simulink model "airspeed_controller16b"  (R2016b)
settings: Solver=FixedStepAuto  StartTime=0.0  StopTime=1000  FixedStep=0.001  RelTol=1e-3
model workspace (MAT data in the model file):
  Cd = 0.18
  SBE_rate_pitch = 0
  climb_max = 5
  g_common = 9.81
  mass_plane = 1.5
  nomThr = 0
  pitch_damping_gain = 0
  pitch_integ_gain = 0.1
  pitch_time_constant = 5
  rou = 1.225
  sink_max = 1
  timeConstThrot = 8
libraries: simulink x2
settings Model: Creator=lee  LastModifiedBy=ls
settings SFSimCC: SimUseLocalCustomCode=on
settings RTWCC: RTWUseLocalCustomCode=on

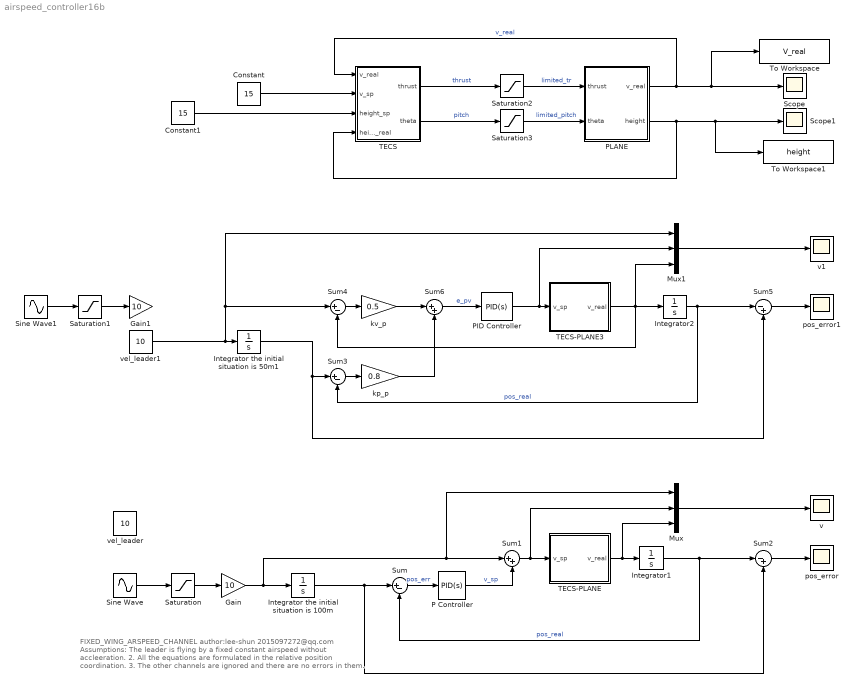
== system airspeed_controller16b ==
  note: FIXED_WING_ARSPEED_CHANNEL
      |
      | author:lee-shun 2015097272@qq.com
      |
      | Assumptions:
      |
      | The leader is flying by a fixed constant airspeed without accleeration.
      | 2. All the equations are formulated in the relative position coordination.
      | 3. The other channels are ignored and there are no errors in them.
  Constant : Constant  Value=15
  Constant1 : Constant  Value=15
  Gain : Gain  Gain=10
  Gain1 : Gain  Gain=10
  Integrator the initial situation is 100m : Integrator  InitialCondition=50  IgnoreLimit=on
  Integrator the initial situation is 50m1 : Integrator  InitialCondition=50  IgnoreLimit=on
  Integrator1 : Integrator
  Integrator2 : Integrator
  Mux : Mux  Inputs=3
  Mux1 : Mux  Inputs=3
  P Controller : simulink/Continuous/PID Controller  Controller=PID  Form=Parallel  TimeDomain=Continuous-time  SampleTime=-1  IntegratorMethod=Forward Euler  FilterMethod=Forward Euler  ControllerParametersSource=internal  P=0.02  I=0  D=0.0  UseFilter=on  N=100  InitialConditionSource=internal  InitialConditionForIntegrator=0  InitialConditionForFilter=0  DifferentiatorICPrevScaledInput=0  ExternalReset=none  TrackingMode=off  Kt=1  LimitOutput=off  UpperSaturationLimit=inf  LowerSaturationLimit=-inf  LinearizeAsGain=on  AntiWindupMode=none  Kb=1  POutMin=[]  POutMax=[]  IOutMin=[]  IOutMax=[]  DOutMin=[]  DOutMax=[]  NOutMin=[]  NOutMax=[]  SumOutMin=[]  SumOutMax=[]  SaturationOutMin=[]  SaturationOutMax=[]  PParamMin=[]  PParamMax=[]  IParamMin=[]  IParamMax=[]  DParamMin=[]  DParamMax=[]  NParamMin=[]  NParamMax=[]  KbParamMin=[]  KbParamMax=[]  KtParamMin=[]  KtParamMax=[]  KbOutMin=[]  KbOutMax=[]  KtOutMin=[]  KtOutMax=[]  IntegratorOutMin=[]  IntegratorOutMax=[]  FilterOutMin=[]  FilterOutMax=[]  SumI1OutMin=[]  SumI1OutMax=[]  SumI2OutMin=[]  SumI2OutMax=[]  SumI3OutMin=[]  SumI3OutMax=[]  SumDOutMin=[]  SumDOutMax=[]  DifferentiatorOutMin=[]  DifferentiatorOutMax=[]  IntegratorContinuousStateAttributes=''  IntegratorStateMustResolveToSignalObject=off  IntegratorRTWStateStorageClass=Auto  FilterContinuousStateAttributes=''  FilterStateMustResolveToSignalObject=off  FilterRTWStateStorageClass=Auto
  PID Controller : simulink/Continuous/PID Controller  Controller=PID  Form=Parallel  TimeDomain=Continuous-time  SampleTime=-1  IntegratorMethod=Forward Euler  FilterMethod=Forward Euler  ControllerParametersSource=internal  P=0.3  I=0.01  D=0  UseFilter=on  N=100  InitialConditionSource=internal  InitialConditionForIntegrator=0  InitialConditionForFilter=0  DifferentiatorICPrevScaledInput=0  ExternalReset=none  TrackingMode=off  Kt=1  LimitOutput=off  UpperSaturationLimit=inf  LowerSaturationLimit=-inf  LinearizeAsGain=on  AntiWindupMode=none  Kb=1  POutMin=[]  POutMax=[]  IOutMin=[]  IOutMax=[]  DOutMin=[]  DOutMax=[]  NOutMin=[]  NOutMax=[]  SumOutMin=[]  SumOutMax=[]  SaturationOutMin=[]  SaturationOutMax=[]  PParamMin=[]  PParamMax=[]  IParamMin=[]  IParamMax=[]  DParamMin=[]  DParamMax=[]  NParamMin=[]  NParamMax=[]  KbParamMin=[]  KbParamMax=[]  KtParamMin=[]  KtParamMax=[]  KbOutMin=[]  KbOutMax=[]  KtOutMin=[]  KtOutMax=[]  IntegratorOutMin=[]  IntegratorOutMax=[]  FilterOutMin=[]  FilterOutMax=[]  SumI1OutMin=[]  SumI1OutMax=[]  SumI2OutMin=[]  SumI2OutMax=[]  SumI3OutMin=[]  SumI3OutMax=[]  SumDOutMin=[]  SumDOutMax=[]  DifferentiatorOutMin=[]  DifferentiatorOutMax=[]  IntegratorContinuousStateAttributes=''  IntegratorStateMustResolveToSignalObject=off  IntegratorRTWStateStorageClass=Auto  FilterContinuousStateAttributes=''  FilterStateMustResolveToSignalObject=off  FilterRTWStateStorageClass=Auto
  PLANE : Subsystem
  Saturation : Saturate  UpperLimit=1  LowerLimit=0.2
  Saturation1 : Saturate  UpperLimit=1  LowerLimit=0.2
  Saturation2 : Saturate  UpperLimit=1  LowerLimit=0  ZeroCross=off
  Saturation3 : Saturate  UpperLimit=pi/4  LowerLimit=-pi/6  ZeroCross=off
  Scope : Scope
  Scope1 : Scope
  Sine Wave : Sin  Frequency=0.1  SampleTime=0
  Sine Wave1 : Sin  Frequency=0.1  SampleTime=0
  Sum : Sum  Inputs=|+-
  Sum1 : Sum  Inputs=|++
  Sum2 : Sum  Inputs=|-+
  Sum3 : Sum  Inputs=|+-
  Sum4 : Sum  Inputs=|+-
  Sum5 : Sum  Inputs=|-+
  Sum6 : Sum  Inputs=|++
  "TECS " : Subsystem
  TECS-PLANE : Subsystem
  TECS-PLANE3 : Subsystem
  To Workspace : ToWorkspace  VariableName=V_real  SaveFormat=Timeseries  SampleTime=-1
  To Workspace1 : ToWorkspace  VariableName=height  SaveFormat=Timeseries  SampleTime=-1
  kp_p : Gain  Gain=0.8
  kv_p : Gain  Gain=0.5
  pos_error : Scope
  pos_error1 : Scope
  v : Scope
  v1 : Scope
  vel_leader : Constant  Value=10
  vel_leader1 : Constant  Value=10
  wires:
  Sum/1 -> P Controller/1  "pos_err"
  Integrator1/1 -> Sum/2, Sum2/1  "pos_real"
  Integrator the initial situation is 100m/1 -> Sum/1, Sum2/2
  TECS-PLANE/1(v_real) -> Mux/3, Integrator1/1
  P Controller/1 -> Sum1/2  "v_sp"
  Sum1/1 -> Mux/2, TECS-PLANE/1(v_sp)
  Sum2/1 -> pos_error/1
  Sine Wave/1 -> Saturation/1
  Saturation/1 -> Gain/1
  Gain/1 -> Mux/1, Sum1/1, Integrator the initial situation is 100m/1
  Mux/1 -> v/1
  Sum5/1 -> pos_error1/1
  Saturation1/1 -> Gain1/1
  Sine Wave1/1 -> Saturation1/1
  TECS-PLANE3/1(v_real) -> Integrator2/1, Mux1/3, Sum4/2
  Integrator2/1 -> Sum5/1, Sum3/2  "pos_real"
  Mux1/1 -> v1/1
  Integrator the initial situation is 50m1/1 -> Sum3/1, Sum5/2
  kv_p/1 -> Sum6/1
  Sum4/1 -> kv_p/1
  Sum3/1 -> kp_p/1
  kp_p/1 -> Sum6/2
  Sum6/1 -> PID Controller/1  "e_pv"
  PID Controller/1 -> TECS-PLANE3/1(v_sp), Mux1/2
  vel_leader1/1 -> Sum4/1, Mux1/1, Integrator the initial situation is 50m1/1
  "TECS "/2("theta ") -> Saturation3/1  "pitch"
  PLANE/1(v_real) -> To Workspace/1, Scope/1, "TECS "/1(v_real)  "v_real"
  PLANE/2(height) -> To Workspace1/1, Scope1/1, "TECS "/4(height_real)
  Saturation3/1 -> PLANE/2(theta)  "limited_pitch"
  Constant/1 -> "TECS "/2(v_sp)
  "TECS "/1(thrust) -> Saturation2/1  "thrust"
  Saturation2/1 -> PLANE/1(thrust)  "limited_tr"
  Constant1/1 -> "TECS "/3(height_sp)

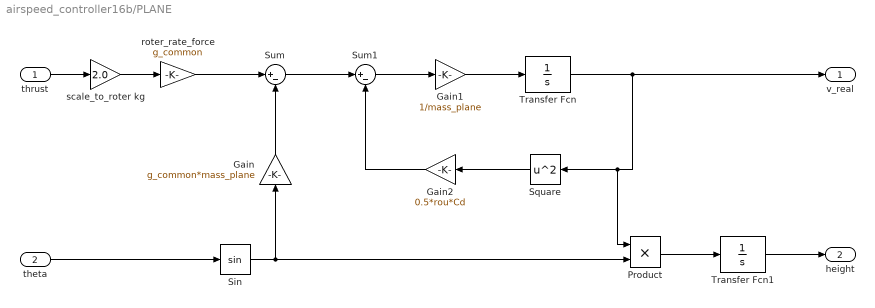
== system airspeed_controller16b/PLANE ==
  thrust : Inport
  theta : Inport  Port=2
  Gain : Gain  Gain=g_common*mass_plane
  Gain1 : Gain  Gain=1/mass_plane
  Gain2 : Gain  Gain=0.5*rou*Cd
  Product : Product
  Sin : Trigonometry
  Square : Math  Operator=square  SaturateOnIntegerOverflow=on
  Sum : Sum  Inputs=|+-
  Sum1 : Sum  Inputs=|+-
  Transfer Fcn : TransferFcn  Denominator=[1 0]
  Transfer Fcn1 : TransferFcn  Denominator=[1 0]
  roter_rate_force : Gain  Gain=g_common
  scale_to_roter kg : Gain  Gain=2.0
  v_real : Outport
  height : Outport  Port=2
  wires:
  thrust/1 -> scale_to_roter kg/1
  scale_to_roter kg/1 -> roter_rate_force/1
  roter_rate_force/1 -> Sum/1
  Gain/1 -> Sum/2
  theta/1 -> Sin/1
  Sin/1 -> Product/2, Gain/1
  Sum/1 -> Sum1/1
  Sum1/1 -> Gain1/1
  Gain1/1 -> Transfer Fcn/1
  Transfer Fcn/1 -> Product/1, Square/1, v_real/1
  Square/1 -> Gain2/1
  Gain2/1 -> Sum1/2
  Product/1 -> Transfer Fcn1/1
  Transfer Fcn1/1 -> height/1

== system airspeed_controller16b/TECS  ==
  v_real : Inport
  v_sp : Inport  Port=2
  height_sp : Inport  Port=3
  height_real : Inport  Port=4
  SBE : Subsystem
  STE : Subsystem
  Subsystem : Subsystem
  Subsystem1 : Subsystem
  Subsystem2 : Subsystem
  thrust : Outport
  "theta " : Outport  Port=2
  wires:
  v_sp/1 -> Subsystem/2(v_sp)
  v_real/1 -> Subsystem2/5(vel_real), Subsystem/1(v_real)
  height_sp/1 -> Subsystem/3(height_sp)
  height_real/1 -> Subsystem/4(height_real)
  Subsystem/1(SPE_sp) -> SBE/1(SPE_sp), STE/1(SPE_sp)
  Subsystem/2(SKE_sp) -> SBE/2(SKE_sp), STE/2(SKE_sp)
  Subsystem/3(SPE_rate_sp) -> SBE/3(SPE_rate_sp), STE/3(SPE_rate_sp)
  Subsystem/4(SKE_rate_sp) -> SBE/4(SKE_rate_sp), STE/4(SKE_rate_sp)
  Subsystem/6(SPE_real) -> SBE/6(SPE_real), STE/6(SPE_real)
  Subsystem/5(SKE_real) -> SBE/5(SKE_real), STE/5(SKE_real)
  Subsystem/7(SKE_rate_real) -> SBE/7(SKE_rate_real), STE/7(SKE_rate_real)
  Subsystem/8(SPE_rate_real) -> SBE/8(SPE_rate_real), STE/8(SPE_rate_real)
  STE/1(STE_real) -> Subsystem1/1(In1)
  STE/2(STE_sp) -> Subsystem1/2(In2)
  STE/3(STE_rate_real) -> Subsystem1/3(In3)
  STE/4(STE_rate_sp) -> Subsystem1/4(In4)
  Subsystem1/1(Out1) -> thrust/1
  SBE/1(SBE_real) -> Subsystem2/1(SBE_real)
  SBE/2(SBE_sp) -> Subsystem2/2(SBE_sp)
  SBE/3(SBE_rate_real) -> Subsystem2/3(SEB_rate_real)
  SBE/4(SBE_rate_sp) -> Subsystem2/4(SEB_rate_sp)
  Subsystem2/1(theta) -> "theta "/1

== system airspeed_controller16b/TECS-PLANE ==
  v_sp : Inport
  PLANE : Subsystem
  Saturation : Saturate  UpperLimit=1  LowerLimit=0  ZeroCross=off
  Scope : Scope
  "TECS " : Subsystem
  v_real : Outport
  wires:
  PLANE/1(v_real) -> v_real/1, "TECS "/2(v_real)  "v_real"
  Saturation/1 -> Scope/1, PLANE/1(thrust)  "limited_tr"
  "TECS "/1(thrust) -> Saturation/1  "thrust"
  v_sp/1 -> "TECS "/1(v_sp)

== system airspeed_controller16b/TECS-PLANE3 ==
  v_sp : Inport
  PLANE : Subsystem
  Saturation : Saturate  UpperLimit=1  LowerLimit=0  ZeroCross=off
  Scope : Scope
  "TECS " : Subsystem
  Zero-Order Hold : ZeroOrderHold  SampleTime=-1
  v_real : Outport
  wires:
  PLANE/1(v_real) -> v_real/1, "TECS "/2(v_real)  "v_real"
  Saturation/1 -> Scope/1, PLANE/1(thrust)  "limited_tr"
  "TECS "/1(thrust) -> Zero-Order Hold/1  "thrust"
  v_sp/1 -> "TECS "/1(v_sp)
  Zero-Order Hold/1 -> Saturation/1

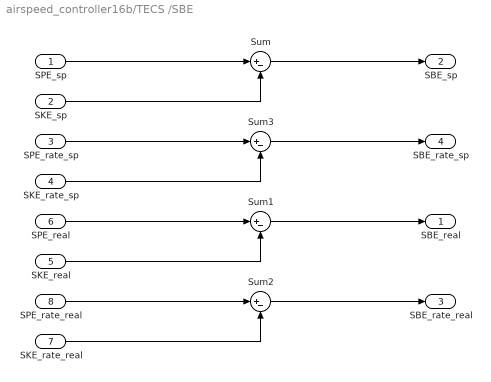
== system airspeed_controller16b/TECS /SBE ==
  SPE_sp : Inport
  SKE_sp : Inport  Port=2
  SPE_rate_sp : Inport  Port=3
  SKE_rate_sp : Inport  Port=4
  SKE_real : Inport  Port=5
  SPE_real : Inport  Port=6
  SKE_rate_real : Inport  Port=7
  SPE_rate_real : Inport  Port=8
  Sum{,1..3} (4 alike) : Sum  Inputs=|+-
  SBE_real : Outport
  SBE_sp : Outport  Port=2
  SBE_rate_real : Outport  Port=3
  SBE_rate_sp : Outport  Port=4
  wires:
  SKE_rate_sp/1 -> Sum3/2
  SKE_sp/1 -> Sum/2
  SPE_rate_sp/1 -> Sum3/1
  SPE_sp/1 -> Sum/1
  Sum/1 -> SBE_sp/1
  SPE_real/1 -> Sum1/1
  SKE_real/1 -> Sum1/2
  Sum1/1 -> SBE_real/1
  Sum3/1 -> SBE_rate_sp/1
  Sum2/1 -> SBE_rate_real/1
  SPE_rate_real/1 -> Sum2/1
  SKE_rate_real/1 -> Sum2/2

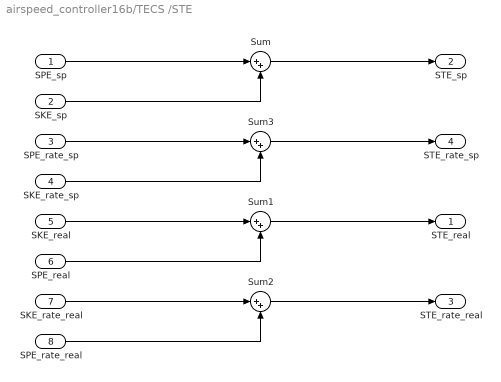
== system airspeed_controller16b/TECS /STE ==
  SPE_sp : Inport
  SKE_sp : Inport  Port=2
  SPE_rate_sp : Inport  Port=3
  SKE_rate_sp : Inport  Port=4
  SKE_real : Inport  Port=5
  SPE_real : Inport  Port=6
  SKE_rate_real : Inport  Port=7
  SPE_rate_real : Inport  Port=8
  Sum{,1..3} (4 alike) : Sum  Inputs=|++
  STE_real : Outport
  STE_sp : Outport  Port=2
  STE_rate_real : Outport  Port=3
  STE_rate_sp : Outport  Port=4
  wires:
  SPE_sp/1 -> Sum/1
  SKE_sp/1 -> Sum/2
  Sum/1 -> STE_sp/1
  SKE_real/1 -> Sum1/1
  Sum1/1 -> STE_real/1
  SPE_real/1 -> Sum1/2
  SKE_rate_real/1 -> Sum2/1
  Sum2/1 -> STE_rate_real/1
  SPE_rate_real/1 -> Sum2/2
  SPE_rate_sp/1 -> Sum3/1
  Sum3/1 -> STE_rate_sp/1
  SKE_rate_sp/1 -> Sum3/2

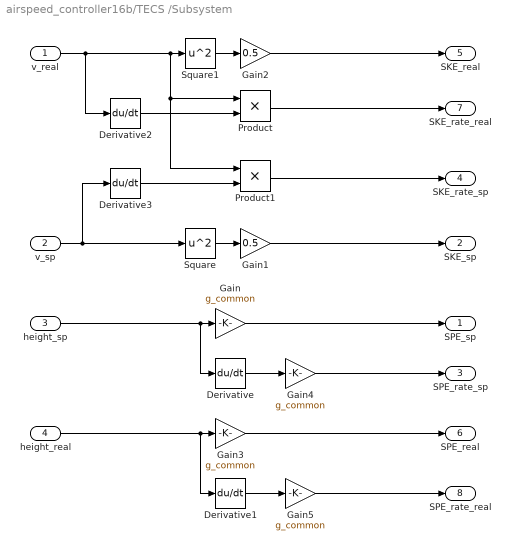
== system airspeed_controller16b/TECS /Subsystem ==
  v_real : Inport
  v_sp : Inport  Port=2
  height_sp : Inport  Port=3
  height_real : Inport  Port=4
  Derivative{,1..3} (4 alike) : Derivative
  Gain{,3..5} (4 alike) : Gain  Gain=g_common
  Gain1 : Gain  Gain=0.5
  Gain2 : Gain  Gain=0.5
  Product : Product
  Product1 : Product
  Square : Math  Operator=square  SaturateOnIntegerOverflow=on
  Square1 : Math  Operator=square  SaturateOnIntegerOverflow=on
  SPE_sp : Outport
  SKE_sp : Outport  Port=2
  SPE_rate_sp : Outport  Port=3
  SKE_rate_sp : Outport  Port=4
  SKE_real : Outport  Port=5
  SPE_real : Outport  Port=6
  SKE_rate_real : Outport  Port=7
  SPE_rate_real : Outport  Port=8
  wires:
  Gain/1 -> SPE_sp/1
  height_sp/1 -> Derivative/1, Gain/1
  Gain1/1 -> SKE_sp/1
  v_sp/1 -> Square/1, Derivative3/1
  Square/1 -> Gain1/1
  Square1/1 -> Gain2/1
  v_real/1 -> Product1/1, Product/1, Square1/1, Derivative2/1
  Gain2/1 -> SKE_real/1
  height_real/1 -> Derivative1/1, Gain3/1
  Gain3/1 -> SPE_real/1
  Gain4/1 -> SPE_rate_sp/1
  Derivative/1 -> Gain4/1
  Gain5/1 -> SPE_rate_real/1
  Derivative1/1 -> Gain5/1
  Product/1 -> SKE_rate_real/1
  Derivative2/1 -> Product/2
  Product1/1 -> SKE_rate_sp/1
  Derivative3/1 -> Product1/2

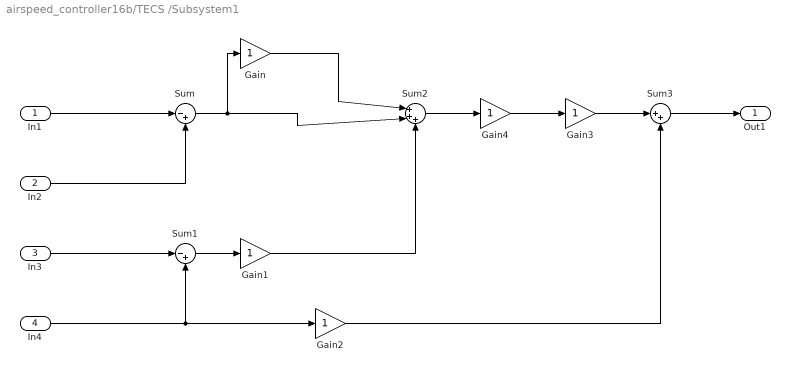
== system airspeed_controller16b/TECS /Subsystem1 ==
  In1 : Inport
  In2 : Inport  Port=2
  In3 : Inport  Port=3
  In4 : Inport  Port=4
  Gain{,1..4} (5 alike) : Gain
  Sum : Sum  Inputs=|-+
  Sum1 : Sum  Inputs=|-+
  Sum2 : Sum  Inputs=|+++
  Sum3 : Sum  Inputs=|++
  Out1 : Outport
  wires:
  Gain3/1 -> Sum3/1
  Sum2/1 -> Gain4/1
  Gain4/1 -> Gain3/1
  In3/1 -> Sum1/1
  Sum3/1 -> Out1/1
  In1/1 -> Sum/1
  In4/1 -> Gain2/1, Sum1/2
  Gain/1 -> Sum2/1
  Sum/1 -> Gain/1, Sum2/2
  In2/1 -> Sum/2
  Sum1/1 -> Gain1/1
  Gain2/1 -> Sum3/2
  Gain1/1 -> Sum2/3

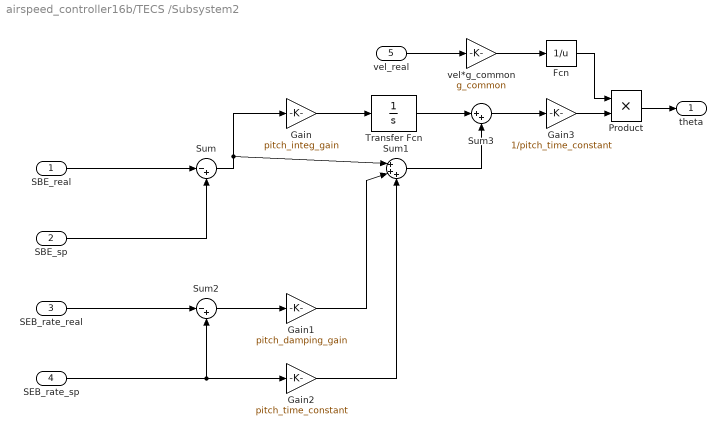
== system airspeed_controller16b/TECS /Subsystem2 ==
  SBE_real : Inport
  SBE_sp : Inport  Port=2
  SEB_rate_real : Inport  Port=3
  SEB_rate_sp : Inport  Port=4
  vel_real : Inport  Port=5
  Fcn : Fcn  Expr=1/u
  Gain : Gain  Gain=pitch_integ_gain
  Gain1 : Gain  Gain=pitch_damping_gain
  Gain2 : Gain  Gain=pitch_time_constant
  Gain3 : Gain  Gain=1/pitch_time_constant
  Product : Product
  Sum : Sum  Inputs=|-+
  Sum1 : Sum  Inputs=|+++
  Sum2 : Sum  Inputs=|-+
  Sum3 : Sum  Inputs=|++
  Transfer Fcn : TransferFcn  Denominator=[1 0]
  vel*g_common : Gain  Gain=g_common
  theta : Outport
  wires:
  Transfer Fcn/1 -> Sum3/1
  Gain3/1 -> Product/2
  Sum3/1 -> Gain3/1
  Sum2/1 -> Gain1/1
  Sum/1 -> Sum1/1, Gain/1
  SBE_sp/1 -> Sum/2
  SEB_rate_sp/1 -> Gain2/1, Sum2/2
  Product/1 -> theta/1
  SEB_rate_real/1 -> Sum2/1
  SBE_real/1 -> Sum/1
  Gain1/1 -> Sum1/2
  Gain2/1 -> Sum1/3
  Sum1/1 -> Sum3/2
  Gain/1 -> Transfer Fcn/1
  vel_real/1 -> vel*g_common/1
  vel*g_common/1 -> Fcn/1
  Fcn/1 -> Product/1

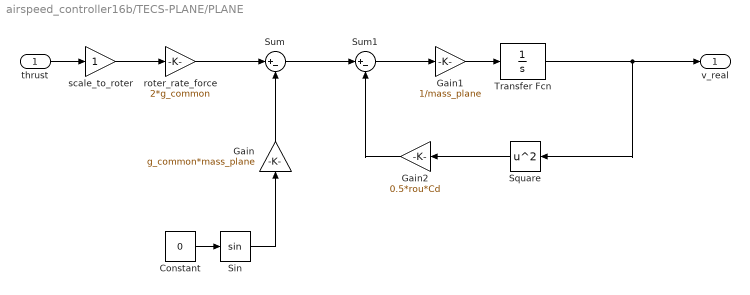
== system airspeed_controller16b/TECS-PLANE/PLANE ==
  thrust : Inport
  Constant : Constant  Value=0
  Gain : Gain  Gain=g_common*mass_plane
  Gain1 : Gain  Gain=1/mass_plane
  Gain2 : Gain  Gain=0.5*rou*Cd
  Sin : Trigonometry
  Square : Math  Operator=square  SaturateOnIntegerOverflow=on
  Sum : Sum  Inputs=|+-
  Sum1 : Sum  Inputs=|+-
  Transfer Fcn : TransferFcn  Denominator=[1 0]
  roter_rate_force : Gain  Gain=2*g_common
  scale_to_roter : Gain
  v_real : Outport
  wires:
  thrust/1 -> scale_to_roter/1
  scale_to_roter/1 -> roter_rate_force/1
  roter_rate_force/1 -> Sum/1
  Gain/1 -> Sum/2
  Constant/1 -> Sin/1
  Sin/1 -> Gain/1
  Sum/1 -> Sum1/1
  Sum1/1 -> Gain1/1
  Gain1/1 -> Transfer Fcn/1
  Transfer Fcn/1 -> Square/1, v_real/1
  Square/1 -> Gain2/1
  Gain2/1 -> Sum1/2

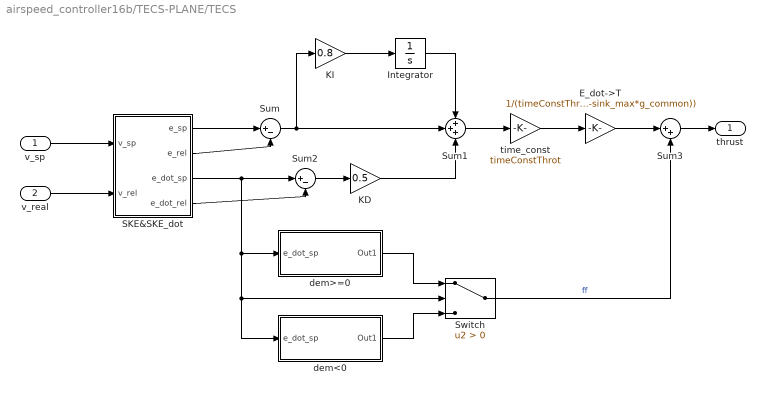
== system airspeed_controller16b/TECS-PLANE/TECS  ==
  v_sp : Inport
  v_real : Inport  Port=2
  E_dot->T : Gain  Gain=1/(timeConstThrot*(climb_max*g_common-sink_max*g_common))
  Integrator : Integrator
  KD : Gain  Gain=0.5
  KI : Gain  Gain=0.8
  SKE&SKE_dot : Subsystem
  Sum : Sum  Inputs=|+-
  Sum1 : Sum  Inputs=+++
  Sum2 : Sum  Inputs=|+-
  Sum3 : Sum  Inputs=|++
  Switch : Switch  Criteria=u2 > Threshold  ZeroCross=off
  dem<0 : Subsystem
  dem>=0 : Subsystem
  time_const : Gain  Gain=timeConstThrot
  thrust : Outport
  wires:
  Sum/1 -> Sum1/2, KI/1
  KI/1 -> Integrator/1
  Integrator/1 -> Sum1/1
  Sum1/1 -> time_const/1
  time_const/1 -> E_dot->T/1
  E_dot->T/1 -> Sum3/1
  v_sp/1 -> SKE&SKE_dot/1(v_sp)
  v_real/1 -> SKE&SKE_dot/2(v_rel)
  SKE&SKE_dot/1(e_sp) -> Sum/1
  SKE&SKE_dot/2(e_rel) -> Sum/2
  SKE&SKE_dot/3(e_dot_sp) -> dem<0/1(e_dot_sp), Switch/2, dem>=0/1(e_dot_sp), Sum2/1
  SKE&SKE_dot/4(e_dot_rel) -> Sum2/2
  Sum2/1 -> KD/1
  KD/1 -> Sum1/3
  Sum3/1 -> thrust/1
  Switch/1 -> Sum3/2  "ff"
  dem>=0/1(Out1) -> Switch/1
  dem<0/1(Out1) -> Switch/3

== system airspeed_controller16b/TECS-PLANE3/PLANE ==
  thrust : Inport
  Constant : Constant  Value=0
  Gain : Gain  Gain=g_common*mass_plane
  Gain1 : Gain  Gain=1/mass_plane
  Gain2 : Gain  Gain=0.5*rou*Cd
  Sin : Trigonometry
  Square : Math  Operator=square  SaturateOnIntegerOverflow=on
  Sum : Sum  Inputs=|+-
  Sum1 : Sum  Inputs=|+-
  Transfer Fcn : TransferFcn  Denominator=[1 0]
  roter_rate_force : Gain  Gain=2*g_common
  scale_to_roter : Gain
  v_real : Outport
  wires:
  thrust/1 -> scale_to_roter/1
  scale_to_roter/1 -> roter_rate_force/1
  roter_rate_force/1 -> Sum/1
  Gain/1 -> Sum/2
  Constant/1 -> Sin/1
  Sin/1 -> Gain/1
  Sum/1 -> Sum1/1
  Sum1/1 -> Gain1/1
  Gain1/1 -> Transfer Fcn/1
  Transfer Fcn/1 -> Square/1, v_real/1
  Square/1 -> Gain2/1
  Gain2/1 -> Sum1/2

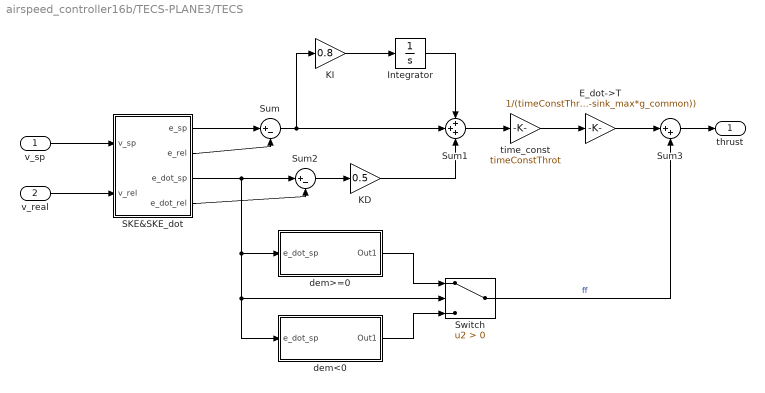
== system airspeed_controller16b/TECS-PLANE3/TECS  ==
  v_sp : Inport
  v_real : Inport  Port=2
  E_dot->T : Gain  Gain=1/(timeConstThrot*(climb_max*g_common-sink_max*g_common))
  Integrator : Integrator
  KD : Gain  Gain=0.5
  KI : Gain  Gain=0.8
  SKE&SKE_dot : Subsystem
  Sum : Sum  Inputs=|+-
  Sum1 : Sum  Inputs=+++
  Sum2 : Sum  Inputs=|+-
  Sum3 : Sum  Inputs=|++
  Switch : Switch  Criteria=u2 > Threshold  ZeroCross=off
  dem<0 : Subsystem
  dem>=0 : Subsystem
  time_const : Gain  Gain=timeConstThrot
  thrust : Outport
  wires:
  Sum/1 -> Sum1/2, KI/1
  KI/1 -> Integrator/1
  Integrator/1 -> Sum1/1
  Sum1/1 -> time_const/1
  time_const/1 -> E_dot->T/1
  E_dot->T/1 -> Sum3/1
  v_sp/1 -> SKE&SKE_dot/1(v_sp)
  v_real/1 -> SKE&SKE_dot/2(v_rel)
  SKE&SKE_dot/1(e_sp) -> Sum/1
  SKE&SKE_dot/2(e_rel) -> Sum/2
  SKE&SKE_dot/3(e_dot_sp) -> dem<0/1(e_dot_sp), Switch/2, dem>=0/1(e_dot_sp), Sum2/1
  SKE&SKE_dot/4(e_dot_rel) -> Sum2/2
  Sum2/1 -> KD/1
  KD/1 -> Sum1/3
  Sum3/1 -> thrust/1
  Switch/1 -> Sum3/2  "ff"
  dem>=0/1(Out1) -> Switch/1
  dem<0/1(Out1) -> Switch/3

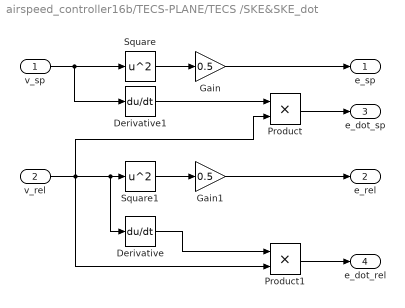
== system airspeed_controller16b/TECS-PLANE/TECS /SKE&SKE_dot ==
  v_sp : Inport
  v_rel : Inport  Port=2
  Derivative : Derivative
  Derivative1 : Derivative
  Gain : Gain  Gain=0.5
  Gain1 : Gain  Gain=0.5
  Product : Product
  Product1 : Product
  Square : Math  Operator=square  SaturateOnIntegerOverflow=on
  Square1 : Math  Operator=square  SaturateOnIntegerOverflow=on
  e_sp : Outport
  e_rel : Outport  Port=2
  e_dot_sp : Outport  Port=3
  e_dot_rel : Outport  Port=4
  wires:
  Square/1 -> Gain/1
  Square1/1 -> Gain1/1
  Gain/1 -> e_sp/1
  v_sp/1 -> Derivative1/1, Square/1
  Gain1/1 -> e_rel/1
  Product/1 -> e_dot_sp/1
  v_rel/1 -> Product1/2, Product/2, Derivative/1, Square1/1
  Product1/1 -> e_dot_rel/1
  Derivative1/1 -> Product/1
  Derivative/1 -> Product1/1

== system airspeed_controller16b/TECS-PLANE/TECS /dem<0 ==
  e_dot_sp : Inport
  Constant : Constant  Value=nomThr
  Gain : Gain  Gain=1/(sink_max*g_common)
  Gain1 : Gain  Gain=nomThr
  Sum : Sum  Inputs=|+-
  Out1 : Outport
  wires:
  Constant/1 -> Sum/1
  e_dot_sp/1 -> Gain/1
  Gain/1 -> Gain1/1
  Gain1/1 -> Sum/2
  Sum/1 -> Out1/1

== system airspeed_controller16b/TECS-PLANE/TECS /dem>=0 ==
  e_dot_sp : Inport
  Constant : Constant  Value=nomThr
  Gain : Gain  Gain=1/(climb_max*g_common)
  Gain1 : Gain  Gain=1-nomThr
  Sum : Sum  Inputs=|++
  Out1 : Outport
  wires:
  Constant/1 -> Sum/1
  e_dot_sp/1 -> Gain/1
  Gain/1 -> Gain1/1
  Gain1/1 -> Sum/2
  Sum/1 -> Out1/1

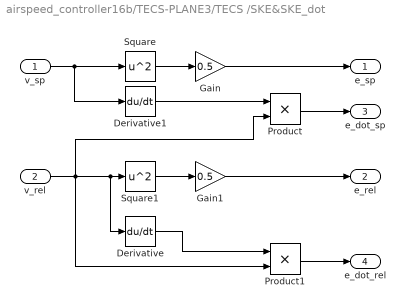
== system airspeed_controller16b/TECS-PLANE3/TECS /SKE&SKE_dot ==
  v_sp : Inport
  v_rel : Inport  Port=2
  Derivative : Derivative
  Derivative1 : Derivative
  Gain : Gain  Gain=0.5
  Gain1 : Gain  Gain=0.5
  Product : Product
  Product1 : Product
  Square : Math  Operator=square  SaturateOnIntegerOverflow=on
  Square1 : Math  Operator=square  SaturateOnIntegerOverflow=on
  e_sp : Outport
  e_rel : Outport  Port=2
  e_dot_sp : Outport  Port=3
  e_dot_rel : Outport  Port=4
  wires:
  Square/1 -> Gain/1
  Square1/1 -> Gain1/1
  Gain/1 -> e_sp/1
  v_sp/1 -> Derivative1/1, Square/1
  Gain1/1 -> e_rel/1
  Product/1 -> e_dot_sp/1
  v_rel/1 -> Product1/2, Product/2, Derivative/1, Square1/1
  Product1/1 -> e_dot_rel/1
  Derivative1/1 -> Product/1
  Derivative/1 -> Product1/1

== system airspeed_controller16b/TECS-PLANE3/TECS /dem<0 ==
  e_dot_sp : Inport
  Constant : Constant  Value=nomThr
  Gain : Gain  Gain=1/(sink_max*g_common)
  Gain1 : Gain  Gain=nomThr
  Sum : Sum  Inputs=|+-
  Out1 : Outport
  wires:
  Constant/1 -> Sum/1
  e_dot_sp/1 -> Gain/1
  Gain/1 -> Gain1/1
  Gain1/1 -> Sum/2
  Sum/1 -> Out1/1

== system airspeed_controller16b/TECS-PLANE3/TECS /dem>=0 ==
  e_dot_sp : Inport
  Constant : Constant  Value=nomThr
  Gain : Gain  Gain=1/(climb_max*g_common)
  Gain1 : Gain  Gain=1-nomThr
  Sum : Sum  Inputs=|++
  Out1 : Outport
  wires:
  Constant/1 -> Sum/1
  e_dot_sp/1 -> Gain/1
  Gain/1 -> Gain1/1
  Gain1/1 -> Sum/2
  Sum/1 -> Out1/1
